simulink model "chap10_2sim"  (Simulink 7.7)
settings: Solver=ode4  SolverMode=SingleTasking  StartTime=0.0  StopTime=20  FixedStep=0.001  RelTol=1e-3
values from neighbouring files (symbols this model uses):
  F1 = 2    [chap10_2int.m]
  F2 = 2.5    [chap10_2int.m]
  F3 = 4    [chap10_2int.m]
  k1 = 0.15    [chap10_2int.m]
  k2 = 0.15    [chap10_2int.m]
  k3 = 0.15    [chap10_2int.m]
  ts = 0.001    [chap10_2int.m]
undefined symbols (not defined in the file or in its folder): den, denc, denz1, denz2, denz3, num, numc, numz1, numz2, numz3
settings Model: Creator=ljk  LastModifiedBy=ljk  ExtModeTrigMode=oneshot  ExtModeArmWhenConnect=off
settings DataIOCC: LimitDataPoints=off  SignalLoggingName=sigsOut
settings OptimizationCC: BooleanDataType=off
settings DebuggingCC: SaveWithParameterizedLinksMsg=none  SignalResolutionControl=TryResolveAllWithWarning  SolverPrmCheckMsg=none  MultiTaskDSMMsg=warning  MultiTaskCondExecSysMsg=none  StrictBusMsg=None
settings HardwareCC: TargetUnknown=on
settings RTWCC: IncludeERTFirstTime=on

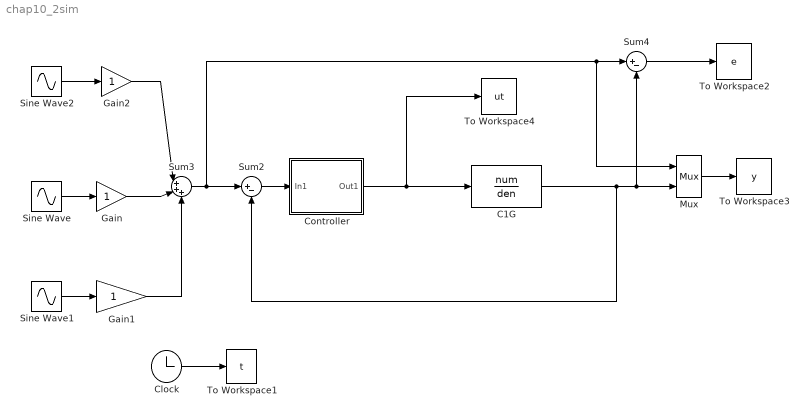
== system chap10_2sim ==
  C1G : DiscreteTransferFcn  Numerator=num  Denominator=den  SampleTime=ts
  Clock : Clock
      settings: Decimation=10
  Controller : Subsystem
  Gain : Gain  SaturateOnIntegerOverflow=on  OutDataTypeStr=Inherit: Same as input  ParamDataTypeStr=Inherit: Same as input
  Gain1 : Gain  SaturateOnIntegerOverflow=on  OutDataTypeStr=Inherit: Same as input  ParamDataTypeStr=Inherit: Same as input
  Gain2 : Gain  SaturateOnIntegerOverflow=on  OutDataTypeStr=Inherit: Same as input  ParamDataTypeStr=Inherit: Same as input
  Mux : Mux  Inputs=2
  Sine Wave : Sin  Frequency=F2*2*pi  SampleTime=ts
  Sine Wave1 : Sin  Frequency=F3*2*pi  Phase=pi/2  SampleTime=ts
  Sine Wave2 : Sin  Frequency=F1*2*pi  SampleTime=ts
  Sum2 : Sum  Inputs=|+-  SaturateOnIntegerOverflow=on  InputSameDT=on  OutDataTypeStr=Inherit: Same as first input
  Sum3 : Sum  Inputs=|+++  SaturateOnIntegerOverflow=on  InputSameDT=on  OutDataTypeStr=Inherit: Same as first input
  Sum4 : Sum  Inputs=|+-  SaturateOnIntegerOverflow=on  InputSameDT=on  OutDataTypeStr=Inherit: Same as first input
  To Workspace1 : ToWorkspace  VariableName=t  SampleTime=-1  SaveFormat=Array
  To Workspace2 : ToWorkspace  VariableName=e  SampleTime=-1  SaveFormat=Array
  To Workspace3 : ToWorkspace  VariableName=y  SampleTime=-1  SaveFormat=Array
  To Workspace4 : ToWorkspace  VariableName=ut  SampleTime=-1  SaveFormat=Array
  wires:
  Mux/1 -> To Workspace3/1
  Sum3/1 -> Sum2/1, Mux/1, Sum4/1
  Sum2/1 -> Controller/1(In1)
  Sum4/1 -> To Workspace2/1
  C1G/1 -> Mux/2, Sum4/2, Sum2/2
  Gain/1 -> Sum3/2
  Sine Wave/1 -> Gain/1
  Sine Wave1/1 -> Gain1/1
  Gain1/1 -> Sum3/3
  Controller/1(Out1) -> C1G/1, To Workspace4/1
  Sine Wave2/1 -> Gain2/1
  Gain2/1 -> Sum3/1
  Clock/1 -> To Workspace1/1

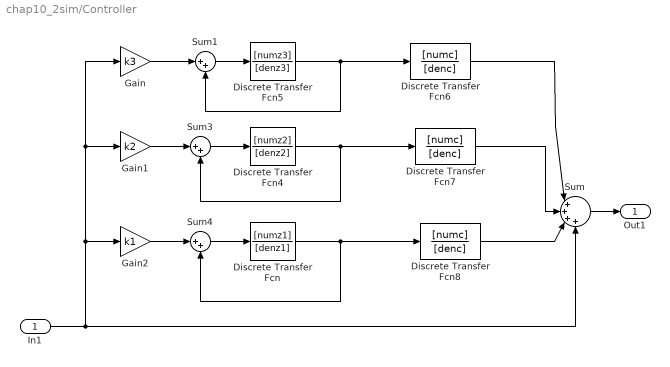
== system chap10_2sim/Controller ==
  In1 : Inport
  Discrete Transfer Fcn : DiscreteTransferFcn  Numerator=[numz1]  Denominator=[denz1]  SampleTime=ts
  Discrete Transfer Fcn4 : DiscreteTransferFcn  Numerator=[numz2]  Denominator=[denz2]  SampleTime=ts
  Discrete Transfer Fcn5 : DiscreteTransferFcn  Numerator=[numz3]  Denominator=[denz3]  SampleTime=ts
  Discrete Transfer Fcn6 : DiscreteTransferFcn  Numerator=[numc]  Denominator=[denc]  SampleTime=ts
  Discrete Transfer Fcn7 : DiscreteTransferFcn  Numerator=[numc]  Denominator=[denc]  SampleTime=ts
  Discrete Transfer Fcn8 : DiscreteTransferFcn  Numerator=[numc]  Denominator=[denc]  SampleTime=ts
  Gain : Gain  Gain=k3  SaturateOnIntegerOverflow=on  OutDataTypeStr=Inherit: Same as input  ParamDataTypeStr=Inherit: Same as input
  Gain1 : Gain  Gain=k2  SaturateOnIntegerOverflow=on  OutDataTypeStr=Inherit: Same as input  ParamDataTypeStr=Inherit: Same as input
  Gain2 : Gain  Gain=k1  SaturateOnIntegerOverflow=on  OutDataTypeStr=Inherit: Same as input  ParamDataTypeStr=Inherit: Same as input
  Sum : Sum  Inputs=|++++  SaturateOnIntegerOverflow=on  InputSameDT=on  OutDataTypeStr=Inherit: Same as first input
  Sum1 : Sum  Inputs=|++  SaturateOnIntegerOverflow=on  InputSameDT=on  OutDataTypeStr=Inherit: Same as first input
  Sum3 : Sum  Inputs=|++  SaturateOnIntegerOverflow=on  InputSameDT=on  OutDataTypeStr=Inherit: Same as first input
  Sum4 : Sum  Inputs=|++  SaturateOnIntegerOverflow=on  InputSameDT=on  OutDataTypeStr=Inherit: Same as first input
  Out1 : Outport
  wires:
  Gain2/1 -> Sum4/1
  Gain1/1 -> Sum3/1
  Sum1/1 -> Discrete Transfer Fcn5/1
  Gain/1 -> Sum1/1
  Sum3/1 -> Discrete Transfer Fcn4/1
  Sum4/1 -> Discrete Transfer Fcn/1
  Sum/1 -> Out1/1
  Discrete Transfer Fcn8/1 -> Sum/3
  Discrete Transfer Fcn7/1 -> Sum/2
  Discrete Transfer Fcn6/1 -> Sum/1
  Discrete Transfer Fcn5/1 -> Sum1/2, Discrete Transfer Fcn6/1
  Discrete Transfer Fcn4/1 -> Sum3/2, Discrete Transfer Fcn7/1
  Discrete Transfer Fcn/1 -> Sum4/2, Discrete Transfer Fcn8/1
  In1/1 -> Sum/4, Gain/1, Gain1/1, Gain2/1
